simulink model "prob_1"  (R2020b)
settings: Solver=VariableStepAuto  StartTime=0.0  StopTime=10.0  RelTol=1e-3
values from neighbouring files (symbols this model uses):
  b = 50    [Problem_1matfile.m]
  K1 = 50    [Problem_1matfile.m]
  k12 = 300    [Problem_1matfile.m]
  M1 = 100    [Problem_1matfile.m]
undefined symbols (not defined in the file or in its folder): m2
settings Model: Creator=Akshay A H  LastModifiedBy=Akshay A H

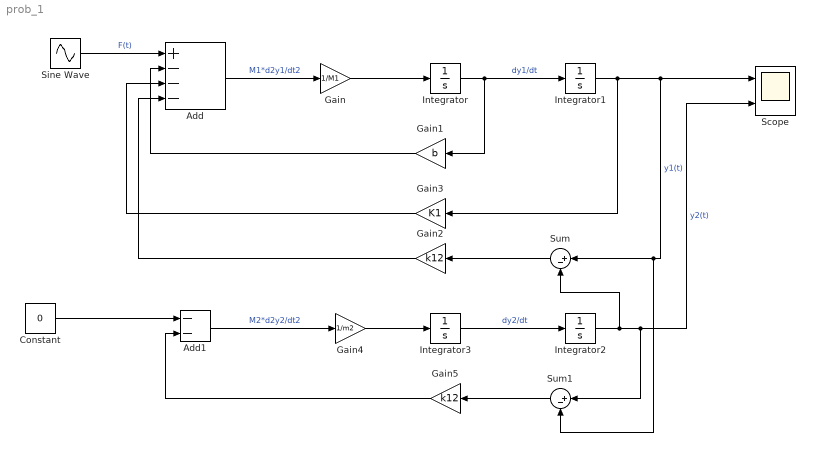
== system prob_1 ==
  Add : Sum  Inputs=+---
  Add1 : Sum  Inputs=--
  Constant : Constant  Value=0
  Gain : Gain  Gain=1/M1
  Gain1 : Gain  Gain=b
  Gain2 : Gain  Gain=k12
  Gain3 : Gain  Gain=K1
  Gain4 : Gain  Gain=1/m2
  Gain5 : Gain  Gain=k12
  Integrator{,1..3} (4 alike) : Integrator
  Scope : Scope  NumInputPorts=2
  Sine Wave : Sin  Amplitude=2  Frequency=10  SampleTime=0
  Sum : Sum  Inputs=|+-
  Sum1 : Sum  Inputs=|+-
  wires:
  Gain4/1 -> Integrator3/1
  Integrator/1 -> Gain1/1, Integrator1/1  "dy1/dt"
  Integrator2/1 -> Sum1/1, Scope/2, Sum/2  "y2(t)"
  Gain1/1 -> Add/2
  Gain/1 -> Integrator/1
  Integrator3/1 -> Integrator2/1  "dy2/dt"
  Add1/1 -> Gain4/1  "M2*d2y2/dt2"
  Constant/1 -> Add1/1
  Gain3/1 -> Add/3
  Add/1 -> Gain/1  "M1*d2y1/dt2"
  Integrator1/1 -> Gain3/1, Sum1/2, Sum/1, Scope/1  "y1(t)"
  Sine Wave/1 -> Add/1  "F(t)"
  Gain5/1 -> Add1/2
  Sum1/1 -> Gain5/1
  Sum/1 -> Gain2/1
  Gain2/1 -> Add/4
